simulink model "MN4008_15_sim"  (R2020b)
settings: Solver=FixedStepAuto  StartTime=0.0  StopTime=10  FixedStep=0.001  RelTol=1e-3
StartFcn:
  | MN4008_15;
StopFcn:
  | %test1;
values from neighbouring files (symbols this model uses):
  J = (J1+J2)*1.5    (= 0.000558)    [MN4008_15.m]
  K = Ke*0.955    (= 0.0252844777062)    [MN4008_15.m]
  Ke = 1/(KV*2*pi/60)*1.414    (= 0.0264758928861)    [MN4008_15.m]
  Kf = 3.5E-6    (= 3.5e-06)    [MN4008_15.m]
  L = 100E-6    (= 0.0001)    [MN4008_15.m]
  R = 98e-3    (= 0.098)    [MN4008_15.m]
libraries: simulink x2
settings Model: Creator=macong  LastModifiedBy=macong
settings DataIOCC: ReturnWorkspaceOutputs=off
settings DebuggingCC: ArithmeticOperatorsInVariantConditions=warning
settings SFSimCC: SimUseLocalCustomCode=off  CustomCodeUndefinedFunction=UseInterfaceOnly
settings RTWCC: RTWUseLocalCustomCode=off

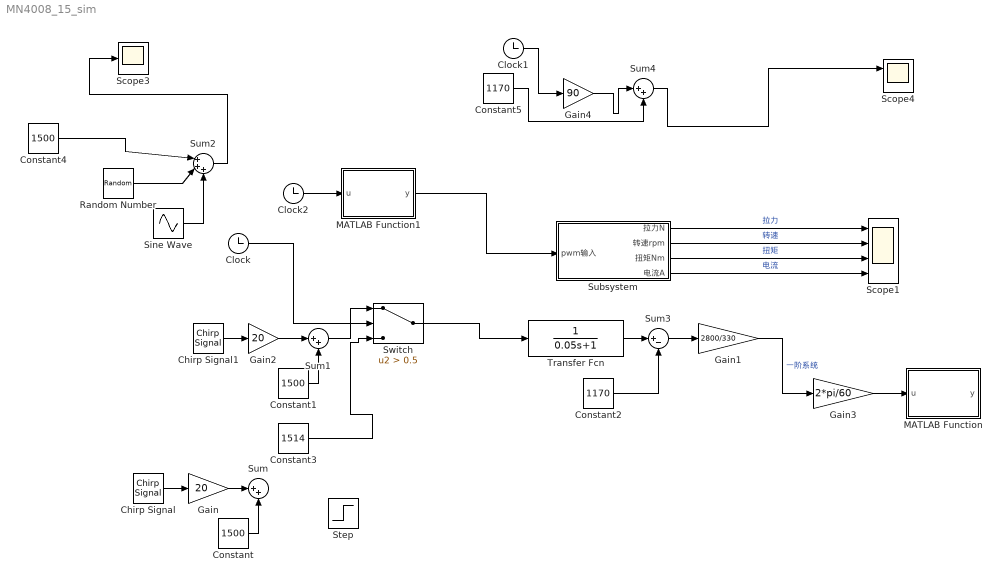
== system MN4008_15_sim ==
  Chirp Signal : simulink/Sources/Chirp Signal  f1=0  T=20  f2=20
  Chirp Signal1 : simulink/Sources/Chirp Signal  f1=0  T=20  f2=20
  Clock : Clock
  Clock1 : Clock
  Clock2 : Clock
  Constant : Constant  Value=1500
  Constant1 : Constant  Value=1500
  Constant2 : Constant  Value=1170
  Constant3 : Constant  Value=1514
  Constant4 : Constant  Value=1500
  Constant5 : Constant  Value=1170
  Gain : Gain  Gain=20
  Gain1 : Gain  Gain=2800/330
  Gain2 : Gain  Gain=20
  Gain3 : Gain  Gain=2*pi/60
  Gain4 : Gain  Gain=90
  MATLAB Function : MATLAB Function  TreatAsAtomicUnit=on
  MATLAB Function1 : MATLAB Function  TreatAsAtomicUnit=on
  Random Number : RandomNumber  Variance=50  SampleTime=0.001
  Scope1 : Scope  NumInputPorts=4
  Scope3 : Scope
  Scope4 : Scope  NumInputPorts=2
  Sine Wave : Sin  Amplitude=10  Frequency=49*2*pi  SampleTime=0.001
  Step : Step  Before=1470  After=1503  SampleTime=0
  Subsystem : Subsystem  mask{pwm_min=1150, pwm_max=1950, V_bat=23.5}
      mask prompts: pwm_min "最低pwm值"; pwm_max "最高pwm值"; V_bat "电池电压"
  Sum : Sum  Inputs=|++
  Sum1 : Sum  Inputs=|++
  Sum2 : Sum  Inputs=|+++
  Sum3 : Sum  Inputs=|+-
  Sum4 : Sum  Inputs=|++
  Switch : Switch  Criteria=u2 > Threshold  Threshold=0.5
  Transfer Fcn : TransferFcn  Denominator=[0.05 1]
  wires:
  Constant/1 -> Sum/2
  Gain/1 -> Sum/1
  Chirp Signal/1 -> Gain/1
  Chirp Signal1/1 -> Gain2/1
  Gain2/1 -> Sum1/1
  Constant1/1 -> Sum1/2
  Sum3/1 -> Gain1/1
  Transfer Fcn/1 -> Sum3/1
  Constant2/1 -> Sum3/2
  Gain1/1 -> Gain3/1  "一阶系统"
  Gain3/1 -> MATLAB Function/1(u)
  Clock/1 -> Switch/2
  Sum1/1 -> Switch/1
  Constant3/1 -> Switch/3
  Switch/1 -> Transfer Fcn/1
  Constant4/1 -> Sum2/1
  Sum2/1 -> Scope3/1
  Random Number/1 -> Sum2/2
  Sine Wave/1 -> Sum2/3
  Clock1/1 -> Gain4/1
  Gain4/1 -> Sum4/1
  Constant5/1 -> Sum4/2
  Sum4/1 -> Scope4/1
  MATLAB Function1/1(y) -> Subsystem/1(pwm输入)
  Subsystem/1(拉力N) -> Scope1/1  "拉力"
  Subsystem/2(转速rpm) -> Scope1/2  "转速"
  Subsystem/3(扭矩Nm) -> Scope1/3  "扭矩"
  Subsystem/4(电流A) -> Scope1/4  "电流"
  Clock2/1 -> MATLAB Function1/1(u)

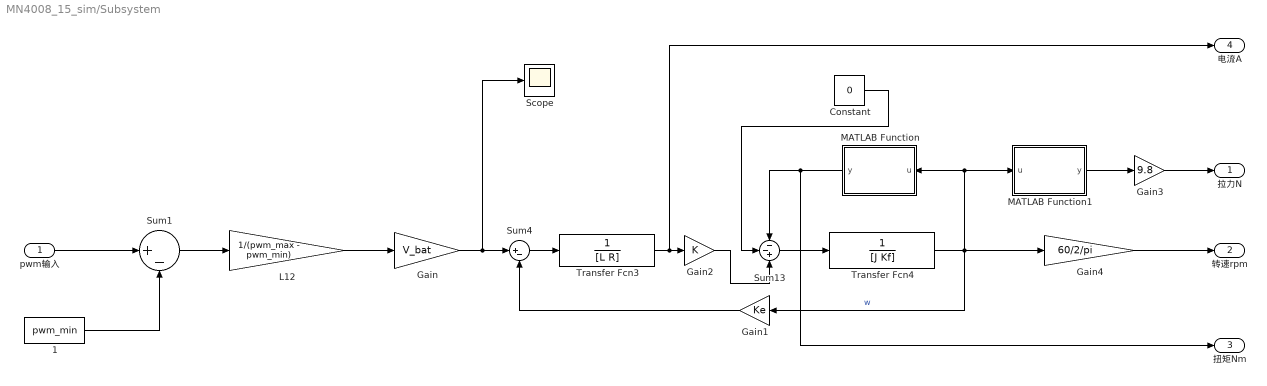
== system MN4008_15_sim/Subsystem ==
  pwm输入 : Inport
  1 : Constant  Value=pwm_min
  Constant : Constant  Value=0
  Gain : Gain  Gain=V_bat
  Gain1 : Gain  Gain=Ke
  Gain2 : Gain  Gain=K
  Gain3 : Gain  Gain=9.8
  Gain4 : Gain  Gain=60/2/pi
  L12 : Gain  Gain=1/(pwm_max - pwm_min)
  MATLAB Function : MATLAB Function  TreatAsAtomicUnit=on
  MATLAB Function1 : MATLAB Function  TreatAsAtomicUnit=on
  Scope : Scope
  Sum1 : Sum  Inputs=|+-
  Sum13 : Sum  Inputs=--+
  Sum4 : Sum  Inputs=|+-
  Transfer Fcn3 : TransferFcn  Denominator=[L R]
  Transfer Fcn4 : TransferFcn  Denominator=[J Kf]
  拉力N : Outport  VectorParamsAs1DForOutWhenUnconnected=off
  转速rpm : Outport  Port=2  VectorParamsAs1DForOutWhenUnconnected=off
  扭矩Nm : Outport  Port=3  VectorParamsAs1DForOutWhenUnconnected=off
  电流A : Outport  Port=4  VectorParamsAs1DForOutWhenUnconnected=off
  wires:
  Sum13/1 -> Transfer Fcn4/1
  Transfer Fcn4/1 -> MATLAB Function1/1(u), MATLAB Function/1(u), Gain1/1, Gain4/1  "w"
  Transfer Fcn3/1 -> 电流A/1, Gain2/1
  Sum4/1 -> Transfer Fcn3/1
  Gain1/1 -> Sum4/2
  Gain4/1 -> 转速rpm/1
  1/1 -> Sum1/2
  Sum1/1 -> L12/1
  pwm输入/1 -> Sum1/1
  MATLAB Function1/1(y) -> Gain3/1
  MATLAB Function/1(y) -> 扭矩Nm/1, Sum13/1
  Gain2/1 -> Sum13/3
  L12/1 -> Gain/1
  Gain/1 -> Scope/1, Sum4/1
  Gain3/1 -> 拉力N/1
  Constant/1 -> Sum13/2

== matlab function MN4008_15_sim/Subsystem/MATLAB Function ==
  data: u input; y output
function y = fcn(u)

% y = (0.0109*u^2 + 0.6552*u)/1000;
% y = (0.0216*u^2 + 0.0374*u)/10000;      %18寸桨力矩曲线，单位nm
y = (0.0911*u^2 - 1.1743*u)/100000;      %tmotor15寸桨力矩曲线，单位nm

== matlab function MN4008_15_sim/Subsystem/MATLAB Function1 ==
  data: u input; y output
function y = fcn(u)

% y = (0.0109*u^2 + 0.6552*u)/1000;
% y = (0.0983*u^2 - 2.6622*u)/10000;      %18寸桨力矩曲线,单位kg
y = (0.0528*u^2 - 4.4005*u)/10000;      %tmotor15寸桨力矩曲线，单位kg

== matlab function MN4008_15_sim/MATLAB Function1 ==
  data: u input; y output
function y = fcn(u)
y = 1150 + 90*floor(u);

end

== matlab function MN4008_15_sim/MATLAB Function ==
  data: u input; y output
function y = fcn(u)

% y = (0.0109*u^2 + 0.6552*u)/1000;
y = (0.0216*u^2 + 0.0374*u)/10000;      %18寸桨力矩曲线
